simulink model "controle_proporcional_onoff_pid"  (R2013a)
settings: Solver=ode45  StartTime=0.0  StopTime=inf  RelTol=1e-3
undefined symbols (not defined in the file): analoginput, analogoutput
libraries: daqlib x2, simulink x2, simulink_extras x1
settings Model: Creator=paulo.costa  LastModifiedBy=paulo.costa

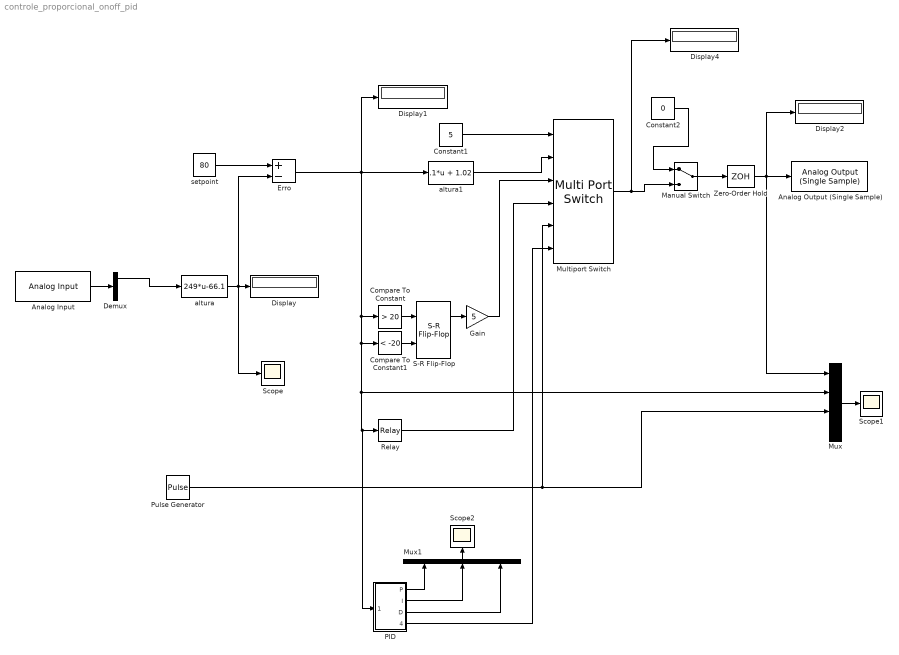
== system controle_proporcional_onoff_pid ==
  Analog Input : daqlib/Analog Input  AcqMode=0  DeviceMenu=nidaq Dev1 (USB-6009)  Device=nidaq Dev1 (USB-6009)  ObjConstructor=analoginput('nidaq','Dev1')  SampleRate=20  ActualRate=20  SamplesPerFrame=2  InputType=SingleEnded  NChannelsSelected=1  Channels=1$0$$2$#0$1$$2$#0$2$$2$#0$3$$2$#0$4$$2$#0$5$$2$#0$6$$2$#0$7$$2$#  NPorts=1 for all hardware channels  DataType=double
      settings: SignalType=Sample-based
  Analog Output (Single Sample) : daqlib/Analog Output (Single Sample)  DeviceMenu=nidaq Dev1 (USB-6009)  Device=nidaq Dev1 (USB-6009)  ObjConstructor=analogoutput('nidaq','Dev1')  NChannelsSelected=1  Channels=1$0$$1$0$#0$1$$1$0$#  NPorts=1 for all hardware channels
  Compare To Constant : simulink/Logic and Bit Operations/Compare To Constant  relop=>  const=20  OutDataTypeStr=boolean
  Compare To Constant1 : simulink/Logic and Bit Operations/Compare To Constant  relop=<  const=-20  OutDataTypeStr=boolean
  Constant1 : Constant  Value=5
  Constant2 : Constant  Value=0
  Demux : Demux  Outputs=2
  Display{,1..2,4} (4 alike) : Display
  Erro : Sum  Inputs=+-
  Gain : Gain  Gain=5
  Manual Switch : ManualSwitch
  Multiport Switch : MultiPortSwitch  Inputs=5
  Mux : Mux
  Mux1 : Mux  Inputs=3
  PID : Subsystem
  Pulse Generator : DiscretePulseGenerator  PulseType=Time based  Amplitude=5  Period=1  PulseWidth=10
  Relay : Relay  OnSwitchValue=20  OffSwitchValue=-20  OnOutputValue=5  OffOutputValue=1
  S-R Flip-Flop : simulink_extras/Flip Flops/S-R Flip-Flop  initial_condition=0
  Scope : Scope
      settings: YMin=157.5  YMax=162.25
  Scope1 : Scope
      settings: TimeRange=10  YMin=-15  YMax=27.5
  Scope2 : Scope
      settings: YMin=-650  YMax=100  SaveName=ScopeData2
  Zero-Order Hold : ZeroOrderHold  SampleTime=.1
  altura : Fcn  Expr=249*u-66.1
  altura1 : Fcn  Expr=.1*u + 1.02
  setpoint : Constant  Value=80
  wires:
  Erro/1 -> altura1/1, Display1/1, PID/1(In1), Relay/1, Mux/2, Compare To Constant1/1, Compare To Constant/1
  Zero-Order Hold/1 -> Mux/1, Display2/1, Analog Output (Single Sample)/1
  altura/1 -> Scope/1, Erro/2, Display/1
  setpoint/1 -> Erro/1
  Compare To Constant1/1 -> S-R Flip-Flop/2
  Compare To Constant/1 -> S-R Flip-Flop/1
  S-R Flip-Flop/1 -> Gain/1
  Mux/1 -> Scope1/1
  Pulse Generator/1 -> Multiport Switch/5, Mux/3
  Gain/1 -> Multiport Switch/3
  Relay/1 -> Multiport Switch/4
  Constant1/1 -> Multiport Switch/1
  Constant2/1 -> Manual Switch/1
  Manual Switch/1 -> Zero-Order Hold/1
  Multiport Switch/1 -> Display4/1, Manual Switch/2
  altura1/1 -> Multiport Switch/2
  Analog Input/1 -> Demux/1
  Demux/1 -> altura/1
  PID/1(P) -> Mux1/1
  PID/2(I) -> Mux1/2
  PID/3(D) -> Mux1/3
  Mux1/1 -> Scope2/1
  PID/4(PID) -> Multiport Switch/6

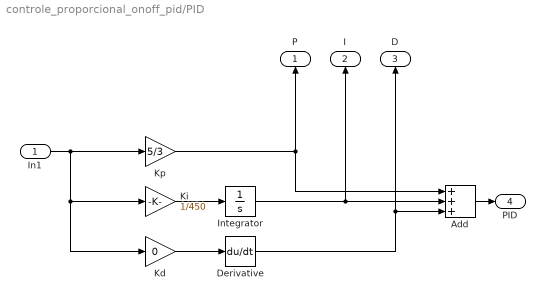
== system controle_proporcional_onoff_pid/PID ==
  In1 : Inport
  Add : Sum  Inputs=+++
  Derivative : Derivative
  Integrator : Integrator
  Kd : Gain  Gain=0
  Ki : Gain  Gain=1/450
  Kp : Gain  Gain=5/3
  P : Outport
  I : Outport  Port=2
  D : Outport  Port=3
  PID : Outport  Port=4
  wires:
  Ki/1 -> Integrator/1
  In1/1 -> Kd/1, Ki/1, Kp/1
  Derivative/1 -> D/1, Add/3
  Add/1 -> PID/1
  Integrator/1 -> I/1, Add/2
  Kp/1 -> P/1, Add/1
  Kd/1 -> Derivative/1
